simulink library "INT_SpdGovSwt_DD"  (R2016b)
settings: Solver=VariableStepAuto  StartTime=0.0  StopTime=10.0  RelTol=1e-3
settings Model: Creator=xinchangran  LastModifiedBy=xinchangran

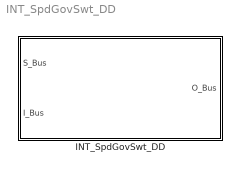
== system INT_SpdGovSwt_DD ==
  INT_SpdGovSwt_DD : Subsystem

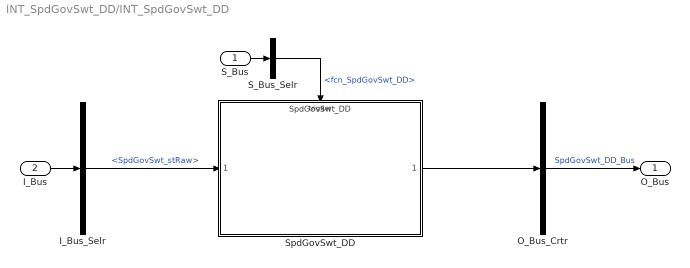
== system INT_SpdGovSwt_DD/INT_SpdGovSwt_DD ==
  S_Bus : Inport
  I_Bus : Inport  Port=2
  I_Bus_Selr : BusSelector  OutputSignals=SpdGovSwt_stRaw
  O_Bus_Crtr : BusCreator  Inputs=1
  S_Bus_Selr : BusSelector  OutputSignals=fcn_SpdGovSwt_DD
  SpdGovSwt_DD : ModelReference  ModelNameDialog=SpdGovSwt_DD  SimulationMode=Normal  ModelReferenceVersion=1.31  TriggerPortName=function  TriggerPortTriggerType=function-call  TriggerPortStatesWhenEnabling=held
  O_Bus : Outport
  wires:
  S_Bus_Selr/1 -> SpdGovSwt_DD/Trigger  "<fcn_SpdGovSwt_DD>"
  S_Bus/1 -> S_Bus_Selr/1
  I_Bus/1 -> I_Bus_Selr/1
  I_Bus_Selr/1 -> SpdGovSwt_DD/1  "<SpdGovSwt_stRaw>"
  O_Bus_Crtr/1 -> O_Bus/1  "SpdGovSwt_DD_Bus"
  SpdGovSwt_DD/1 -> O_Bus_Crtr/1
